simulink model "Non_isolated_Buck_Boost_Converter_IdealCase"  (R2021a)
settings: Solver=VariableStepAuto  StartTime=0.0  StopTime=0.1  RelTol=1e-3
libraries: spsVoltageMeasurementLib x6, spsCurrentMeasurementLib x5, spsSeriesRLCBranchLib x3, spsDiodeLib x1, spsMosfetLib x1, spsDCVoltageSourceLib x1, spspowerguiLib x1
settings Model: NumberOfSteps=2  Creator=EREN-PC  LastModifiedBy=EREN-PC

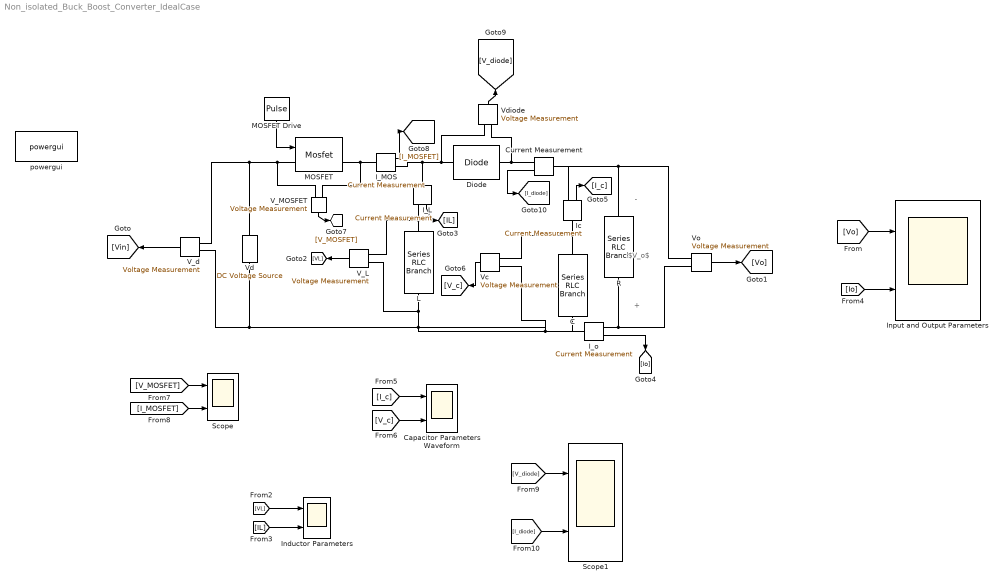
== system Non_isolated_Buck_Boost_Converter_IdealCase ==
  note: -
  note: +
  note: $V_o$
  C : spsSeriesRLCBranchLib/Series RLC Branch  LConnTagsString=__new0  RConnTagsString=__new0  BranchType=C  Resistance=1  Inductance=1e-3  SetiL0=off  InitialCurrent=0  Capacitance=9e-4  Setx0=off  InitialVoltage=0  Measurements=None
  Capacitor Parameters Waveform : Scope  NumInputPorts=2
  Current Measurement : spsCurrentMeasurementLib/Current Measurement  PhasorSimulation=off  OutputType=Complex  PSBequivalent=0
  Diode : spsDiodeLib/Diode  Ron=0.001  Lon=0  Vf=0.8  IC=0  UseSnubber=0  Rs=500  Cs=250e-9  Measurements=off
  I_L : spsCurrentMeasurementLib/Current Measurement  PhasorSimulation=off  OutputType=Complex  PSBequivalent=0
  I_MOS : spsCurrentMeasurementLib/Current Measurement  PhasorSimulation=off  OutputType=Complex  PSBequivalent=0
  I_o : spsCurrentMeasurementLib/Current Measurement  PhasorSimulation=off  OutputType=Complex  PSBequivalent=0
  Ic : spsCurrentMeasurementLib/Current Measurement  PhasorSimulation=off  OutputType=Complex  PSBequivalent=0
  Inductor Parameters : Scope  NumInputPorts=2
  Input and Output Parameters : Scope  NumInputPorts=2
  L : spsSeriesRLCBranchLib/Series RLC Branch  LConnTagsString=__new0  RConnTagsString=__new0  BranchType=L  Resistance=1  Inductance=1.38e-3  SetiL0=off  InitialCurrent=0  Capacitance=1e-6  Setx0=off  InitialVoltage=0  Measurements=None
  MOSFET : spsMosfetLib/Mosfet  Ron=0.1  Lon=0  Rd=0.01  Vfd=0  IC=0  Rs=1e5  Cs=inf  Measurements=on
  MOSFET Drive : DiscretePulseGenerator  PulseType=Time based  Period=20e-6  PulseWidth=45
  R : spsSeriesRLCBranchLib/Series RLC Branch  LConnTagsString=__new0  RConnTagsString=__new0  BranchType=R  Resistance=6  Inductance=1e-3  SetiL0=off  InitialCurrent=0  Capacitance=1e-6  Setx0=off  InitialVoltage=0  Measurements=None
  Scope : Scope  NumInputPorts=2
  Scope1 : Scope  NumInputPorts=2
  V_L : spsVoltageMeasurementLib/Voltage Measurement  PhasorSimulation=off  OutputType=Complex  PSBequivalent=0
  V_MOSFET : spsVoltageMeasurementLib/Voltage Measurement  PhasorSimulation=off  OutputType=Complex  PSBequivalent=0
  V_d : spsVoltageMeasurementLib/Voltage Measurement  PhasorSimulation=off  OutputType=Complex  PSBequivalent=0
  Vc : spsVoltageMeasurementLib/Voltage Measurement  PhasorSimulation=off  OutputType=Complex  PSBequivalent=0
  Vd : spsDCVoltageSourceLib/DC Voltage Source  Amplitude=16  Measurements=None
  Vdiode : spsVoltageMeasurementLib/Voltage Measurement  PhasorSimulation=off  OutputType=Complex  PSBequivalent=0
  Vo : spsVoltageMeasurementLib/Voltage Measurement  PhasorSimulation=off  OutputType=Complex  PSBequivalent=0
  powergui : spspowerguiLib/powergui  Priority=1  SimulationMode=Continuous  SampleTime=50e-6  frequency=60  Iterations=50  frequencyindice=0  Pbase=100e6  ErrMax=1e-4  UnitsV=kV  UnitsW=MW  buscounter=0  FunctionMessages=off  echomessages=off  EnableUseOfTLC=off  CurrentSourceSwitches=off  DisableSnubberDevices=off  DisableRonSwitches=off  DisableVfSwitches=off  DisplayEquations=off  AutomaticDiscreteSolvers=off  SolverType=Tustin/Backward Euler (TBE)  Interpol=off  ExternalGateDelay=off  methode=off  Ts=100  x0status=blocks  SPID=on  SwTol=0  HookPort=off  NonlinearTolerance=1e-4  nMaxIteration=100  ContinueOnMaxIteration=off  RestoreLinks=warning  ResistiveCurrentMeasurement=off  Frange=[0:2:500]  Ylog=off  Xlog=on  ShowGrid=off  save=off  variable=ZData  structure=0  ZoomFFT=off  StartTime=0.0  cycles=1  DisplayStyle=1  fundamental=60  FreqAxis=off  MaxFrequency=1000  frequencyindicesteady=1  RmsSteady=1  display=off
  wires:
  MOSFET Drive/1 -> MOSFET/1
  Vo/1 -> [Vo]
  [Vo] -> Input and Output Parameters/1
  V_d/1 -> [Vin]
  V_L/1 -> [VL]
  [VL] -> Inductor Parameters/1
  [IL] -> Inductor Parameters/2
  I_L/1 -> [IL]
  I_o/1 -> [Io]
  [Io] -> Input and Output Parameters/2
  [I_c] -> Capacitor Parameters Waveform/1
  Ic/1 -> [I_c]
  Vc/1 -> [V_c]
  [V_c] -> Capacitor Parameters Waveform/2
  V_MOSFET/1 -> [V_MOSFET]
  [V_MOSFET] -> Scope/1
  I_MOS/1 -> [I_MOSFET]
  [I_MOSFET] -> Scope/2
  Vdiode/1 -> [V_diode]
  [V_diode] -> Scope1/1
  [I_diode] -> Scope1/2
  Current Measurement/1 -> [I_diode]
  connections:
  Vd/RConn1 -- V_d/LConn1 -- V_MOSFET/LConn1 -- MOSFET/LConn1
  L/RConn1 -- V_L/LConn2 -- C/RConn1 -- I_o/LConn1 -- Vc/LConn1 -- Vd/LConn1 -- V_d/LConn2
  I_L/RConn1 -- V_L/LConn1 -- L/LConn1
  Diode/RConn1 -- Vdiode/LConn2 -- I_L/LConn1 -- I_MOS/RConn1
  I_o/RConn1 -- Vo/LConn1 -- R/RConn1
  Ic/LConn1 -- Vc/LConn2 -- C/LConn1
  V_MOSFET/LConn2 -- MOSFET/RConn1 -- I_MOS/LConn1
  Diode/LConn1 -- Current Measurement/RConn1 -- Vdiode/LConn1
  R/LConn1 -- Current Measurement/LConn1 -- Ic/RConn1 -- Vo/LConn2
